simulink model "cartpolesimulation"  (R2016a)
settings: Solver=VariableStepAuto  StartTime=0.0  StopTime=10.0  RelTol=1e-3
values from neighbouring files (symbols this model uses):
  g = 9.8    [CartPoleLQR.m]    (also in CartPolePID.m; CartPoleStateSpaceModel.m)
  m = 0.1    [CartPoleLQR.m]    (also in CartPolePID.m; CartPoleStateSpaceModel.m)
  M = 1    [CartPoleLQR.m]    (also in CartPolePID.m; CartPoleStateSpaceModel.m)
undefined symbols (not defined in the file or in its folder): L
libraries: simulink x1
settings Model: Creator=spshetty  LastModifiedBy=spshetty
settings DataIOCC: SaveState=on

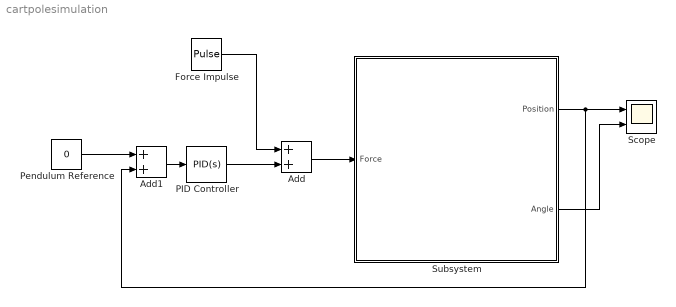
== system cartpolesimulation ==
  Add : Sum
  Add1 : Sum
  Force Impulse : DiscretePulseGenerator  PulseType=Time based  Period=10  PulseWidth=5
  PID Controller : simulink/Continuous/PID Controller  Controller=PID  TimeDomain=Continuous-time  SampleTime=-1  IntegratorMethod=Forward Euler  FilterMethod=Forward Euler  Form=Parallel  UseFilter=on  ControllerParametersSource=internal  P=0.9  I=0  D=0  N=100  InitialConditionSource=internal  InitialConditionForIntegrator=0  InitialConditionForFilter=0  ExternalReset=none  LimitOutput=off  UpperSaturationLimit=inf  LowerSaturationLimit=-inf  LinearizeAsGain=on  AntiWindupMode=none  Kb=1  TrackingMode=off  Kt=1  PParamMin=[]  PParamMax=[]  IParamMin=[]  IParamMax=[]  DParamMin=[]  DParamMax=[]  NParamMin=[]  NParamMax=[]  KbParamMin=[]  KbParamMax=[]  KtParamMin=[]  KtParamMax=[]  POutMin=[]  POutMax=[]  IOutMin=[]  IOutMax=[]  DOutMin=[]  DOutMax=[]  NOutMin=[]  NOutMax=[]  KbOutMin=[]  KbOutMax=[]  KtOutMin=[]  KtOutMax=[]  IntegratorOutMin=[]  IntegratorOutMax=[]  FilterOutMin=[]  FilterOutMax=[]  SumOutMin=[]  SumOutMax=[]  SumI1OutMin=[]  SumI1OutMax=[]  SumI2OutMin=[]  SumI2OutMax=[]  SumI3OutMin=[]  SumI3OutMax=[]  SumDOutMin=[]  SumDOutMax=[]  SaturationOutMin=[]  SaturationOutMax=[]  IntegratorContinuousStateAttributes=''  IntegratorStateMustResolveToSignalObject=off  IntegratorRTWStateStorageClass=Auto  FilterContinuousStateAttributes=''  FilterStateMustResolveToSignalObject=off  FilterRTWStateStorageClass=Auto  DifferentiatorICPrevScaledInput=0  DifferentiatorOutMin=[]  DifferentiatorOutMax=[]
  Pendulum Reference : Constant  Value=0
  Scope : Scope  NumInputPorts=2
  Subsystem : Subsystem
  wires:
  Add/1 -> Subsystem/1(Force)
  PID Controller/1 -> Add/2
  Force Impulse/1 -> Add/1
  Add1/1 -> PID Controller/1
  Subsystem/1(Position) -> Scope/1, Add1/2
  Subsystem/2(Angle) -> Scope/2
  Pendulum Reference/1 -> Add1/1

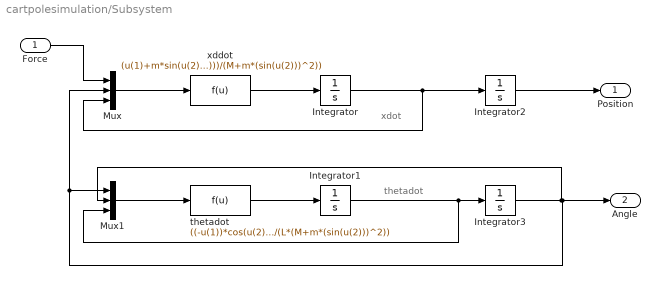
== system cartpolesimulation/Subsystem ==
  note: thetadot
  note: xdot
  Force : Inport
  Integrator : Integrator  ContinuousStateAttributes='xdot'
  Integrator1 : Integrator  InitialCondition=pi  ContinuousStateAttributes='thetadot'
  Integrator2 : Integrator  ContinuousStateAttributes='x'
  Integrator3 : Integrator  ContinuousStateAttributes='theta'
  Mux : Mux  Inputs=3
  Mux1 : Mux  Inputs=3
  thetadot : Fcn  Expr=((-u(1))*cos(u(2))-m*L*((u(3))^2)*sin(u(2))*cos(u(2))+(M+m)*g*sin(u(2)))/(L*(M+m*(sin(u(2)))^2))
  xddot : Fcn  Expr=(u(1)+m*sin(u(2))*(L*((u(3))^2)-g*cos(u(2)))/(M+m*(sin(u(2)))^2))
  Position : Outport
  Angle : Outport  Port=2
  wires:
  Mux1/1 -> thetadot/1
  Integrator3/1 -> Angle/1, Mux1/1, Mux/2, Mux1/2
  Mux/1 -> xddot/1
  thetadot/1 -> Integrator1/1
  Integrator1/1 -> Mux1/3, Integrator3/1
  Integrator/1 -> Mux/3, Integrator2/1
  Integrator2/1 -> Position/1
  Force/1 -> Mux/1
  xddot/1 -> Integrator/1
